simulink model "Battery_module"  (R2021a)
settings: Solver=VariableStepAuto  StartTime=0.0  StopTime=1.5  RelTol=1e-3
undefined symbols (not defined in the file or in its folder): Ion, Lithium
libraries: spsOnDelayLib x2, spsBatteryLib x2, spsDCVoltageSourceLib x1, spsSeriesRLCBranchLib x1, pid_lib x1, eePwmGenerator x1, spsMeanLib x1, spsUniversalBridgeLib x1, spsVoltageMeasurementLib x1, spspowerguiLib x1, SignalEditorBlockLib x1
settings Model: Creator=XieWHirlwind_TB  LastModifiedBy=XieWHirlwind_TB

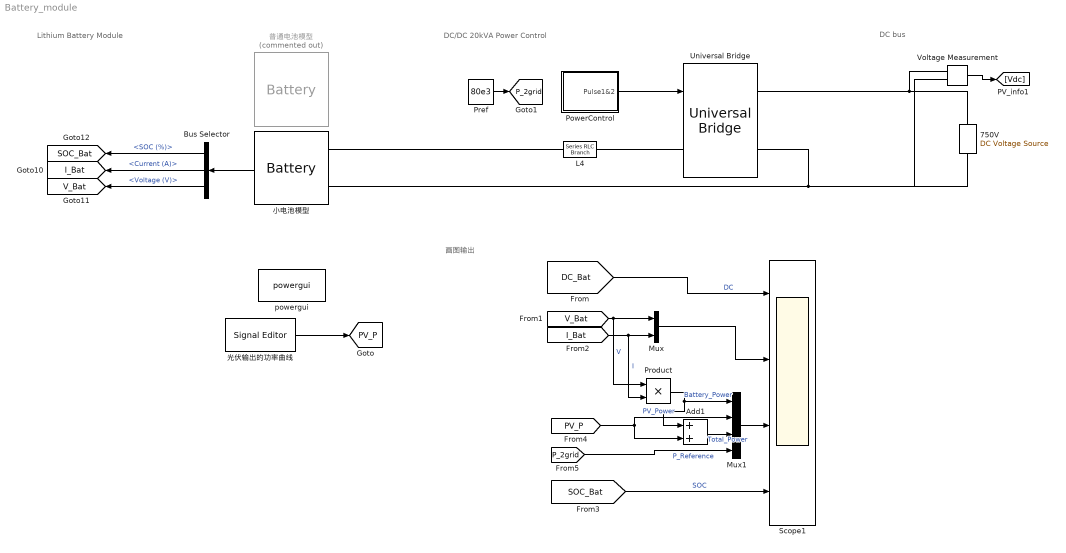
== system Battery_module ==
  note: 画图输出
  note: DC/DC 20kVA Power Control
  note: Lithium Battery Module
  note: DC bus
  750V : spsDCVoltageSourceLib/DC Voltage Source  Amplitude=750  Measurements=None
  Add1 : Sum
  Bus Selector : BusSelector  OutputSignals=SOC (%),Current (A),Voltage (V)
  L4 : spsSeriesRLCBranchLib/Series RLC Branch  LConnTagsString=__new0  RConnTagsString=__new0  BranchType=RL  Resistance=0.001  Inductance=1e-3  SetiL0=off  InitialCurrent=0  Capacitance=1e-6  Setx0=off  InitialVoltage=0  Measurements=None
  Mux : Mux  Inputs=2
  Mux1 : Mux
  PowerControl : Subsystem
  Pref : Constant  Value=80e3
  Product : Product
  Scope1 : Scope  NumInputPorts=4
  Universal Bridge : spsUniversalBridgeLib/Universal Bridge  Arms=1  SnubberResistance=1e5  SnubberCapacitance=inf  Device=IGBT / Diodes  Ron=1e-3  Lon=0  ForwardVoltages="[0.7  0.7]"  ForwardVoltage=0  GTOparameters=[ 10e-6 , 20e-6 ]  IGBTparameters=[ 1e-6 , 2e-6 ]  Measurements=None  Measurements_2=None  converterType=Rectifier
  Voltage Measurement : spsVoltageMeasurementLib/Voltage Measurement  PhasorSimulation=off  OutputType=Complex  PSBequivalent=0
  powergui : spspowerguiLib/powergui  Priority=1  SimulationMode=Discrete  SampleTime=2e-6  frequency=60  Iterations=50  frequencyindice=0  Pbase=100e6  ErrMax=1e-4  UnitsV=kV  UnitsW=MW  buscounter=0  FunctionMessages=off  echomessages=off  EnableUseOfTLC=off  CurrentSourceSwitches=off  DisableSnubberDevices=off  DisableRonSwitches=off  DisableVfSwitches=off  DisplayEquations=off  AutomaticDiscreteSolvers=off  SolverType=Tustin/Backward Euler (TBE)  Interpol=off  ExternalGateDelay=off  methode=off  Ts=100  x0status=blocks  SPID=on  SwTol=0  HookPort=off  NonlinearTolerance=1e-4  nMaxIteration=100  ContinueOnMaxIteration=off  RestoreLinks=warning  ResistiveCurrentMeasurement=off  Frange=[0:2:500]  Ylog=off  Xlog=on  ShowGrid=off  save=off  variable=ZData  structure=0  ZoomFFT=off  StartTime=0.0  cycles=1  DisplayStyle=1  fundamental=60  FreqAxis=off  MaxFrequency=1000  frequencyindicesteady=1  RmsSteady=1  display=off
  光伏输出的功率曲线 : SignalEditorBlockLib/Signal Editor  FileName=PV_Power_1.mat  ActiveScenario=InRatedPower  ActiveSignal=PV_Power  IsBus=off  OutputBusObjectStr=Bus: BusObject  SampleTime=0  ZeroCross=off  OutputAfterFinalValue=Setting to zero  Unit=inherit  PreserveSignalName=on
  小电池模型 : spsBatteryLib/Battery  BatType=Lithium-Ion  ShowTempParam=off  ThermalPreset=no  ShowAgeParam=off  NomV=640  NomQ=62.5/1000  SOC=50  Batt_Tr=30  PresetModel=off  MaxQ=62.5/100000  MinV=480  FullV=744.9518  Dis_rate=27.1739  R=0.1024  Normal_OP=56.5217/100000  expZone="[691.4469      3.070652/100000]"  current=[6.5 13 32.5]  Units=Time  Tci=20  NomT=20  T2=-30  MaxQ2=4.8  FullV2=7.1  Normal_OP2=5.655  expZone2="[6.58           1]"  Rca=0.6  ti=2000  Dp=0  Neq0=0  Tsim=1e6  Ta1=25  Qeol=5.4*0.9  Reol=0.013333*1.2  Char_age=[2.3478, 3]  Dis_age=[2.3478, 10]  N1=1500  N2=10500  N3=1000  N4=1400  Ta2=45  N5=950
  普通电池模型 : spsBatteryLib/Battery  Commented=on  BatType=Lithium-Ion  ShowTempParam=off  ThermalPreset=no  ShowAgeParam=off  NomV=640  NomQ=62.5  SOC=50  Batt_Tr=30  PresetModel=on  MaxQ=62.5  MinV=480  FullV=744.9518  Dis_rate=27.1739  R=0.1024  Normal_OP=56.5217  expZone="[691.4469      3.070652]"  current=[6.5 13 32.5]  Units=Time  Tci=20  NomT=20  T2=-30  MaxQ2=4.8  FullV2=7.1  Normal_OP2=5.655  expZone2="[6.58           1]"  Rca=0.6  ti=2000  Dp=0  Neq0=0  Tsim=1e6  Ta1=25  Qeol=5.4*0.9  Reol=0.013333*1.2  Char_age=[2.3478, 3]  Dis_age=[2.3478, 10]  N1=1500  N2=10500  N3=1000  N4=1400  Ta2=45  N5=950
  tag scope: I_Bat=global, PV_P=global, P_2grid=global, SOC_Bat=global, V_Bat=global
  wires:
  Bus Selector/3 -> [V_Bat]  "<Voltage (V)>"
  小电池模型/1 -> Bus Selector/1
  Bus Selector/1 -> [SOC_Bat]  "<SOC (%)>"
  Bus Selector/2 -> [I_Bat]  "<Current (A)>"
  Voltage Measurement/1 -> [Vdc]
  光伏输出的功率曲线/1 -> [PV_P]
  [DC_Bat] -> Scope1/1  "DC"
  [V_Bat] -> Mux/1, Product/1  "V"
  [I_Bat] -> Product/2, Mux/2  "I"
  [SOC_Bat] -> Scope1/4  "SOC"
  Mux/1 -> Scope1/2
  [PV_P] -> Add1/2, Mux1/2  "PV_Power"
  Mux1/1 -> Scope1/3
  Product/1 -> Add1/1, Mux1/1  "Battery_Power"
  Add1/1 -> Mux1/3  "Total_Power"
  PowerControl/1(Pulse1&2) -> Universal Bridge/1
  Pref/1 -> [P_2grid]
  [P_2grid] -> Mux1/4  "P_Reference"
  connections:
  750V/LConn1 -- Voltage Measurement/LConn2 -- 小电池模型/LConn2 -- Universal Bridge/RConn2
  Universal Bridge/LConn1 -- L4/RConn1
  小电池模型/LConn1 -- L4/LConn1
  Universal Bridge/RConn1 -- 750V/RConn1 -- Voltage Measurement/LConn1

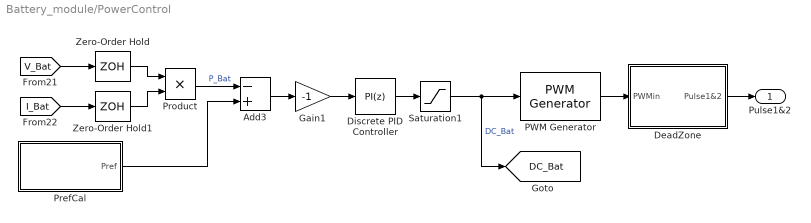
== system Battery_module/PowerControl ==
  Add3 : Sum  Inputs=-+
  DeadZone : Subsystem
  Discrete PID Controller : pid_lib/PID Controller  Controller=PI  Form=Parallel  TimeDomain=Discrete-time  UseExternalTs=off  SampleTime=1e-4  IntegratorMethod=Forward Euler  FilterMethod=Forward Euler  ControllerParametersSource=internal  P=2e-6  I=2e-3  D=0  UseFilter=on  N=100  TunerSelectOption=Transfer Function Based (PID Tuner App)  InitialConditionSource=internal  InitialConditionForIntegrator=0.8  InitialConditionForFilter=0  DifferentiatorICPrevScaledInput=0  ExternalReset=none  TrackingMode=off  Kt=1  LimitOutput=off  SatLimitsSource=internal  UpperSaturationLimit=1  LowerSaturationLimit=0  LinearizeAsGain=off  AntiWindupMode=none  Kb=1  POutMin=[]  POutMax=[]  IOutMin=[]  IOutMax=[]  DOutMin=[]  DOutMax=[]  NOutMin=[]  NOutMax=[]  SumOutMin=[]  SumOutMax=[]  SaturationOutMin=[]  SaturationOutMax=[]  PParamMin=[]  PParamMax=[]  IParamMin=[]  IParamMax=[]  DParamMin=[]  DParamMax=[]  NParamMin=[]  NParamMax=[]  KbParamMin=[]  KbParamMax=[]  KtParamMin=[]  KtParamMax=[]  KbOutMin=[]  KbOutMax=[]  KtOutMin=[]  KtOutMax=[]  IntegratorOutMin=[]  IntegratorOutMax=[]  FilterOutMin=[]  FilterOutMax=[]  SumI1OutMin=[]  SumI1OutMax=[]  SumI2OutMin=[]  SumI2OutMax=[]  SumI3OutMin=[]  SumI3OutMax=[]  SumI4OutMin=[]  SumI4OutMax=[]  SumDOutMin=[]  SumDOutMax=[]  DifferentiatorOutMin=[]  DifferentiatorOutMax=[]  FilterDiffOutCoefMin=[]  FilterDiffOutCoefMax=[]  ReciprocalOutMin=[]  ReciprocalOutMax=[]  SumDenOutMin=[]  SumDenOutMax=[]  SumNumOutMin=[]  SumNumOutMax=[]  DivideOutMin=[]  DivideOutMax=[]  UdiffTsProdOutMin=[]  UdiffTsProdOutMax=[]  NTsProdOutMin=[]  NTsProdOutMax=[]  UintegralTsProdOutMin=[]  UintegralTsProdOutMax=[]  UngainTsProdOutMin=[]  UngainTsProdOutMax=[]  IntegratorContinuousStateAttributes=''  IntegratorStateMustResolveToSignalObject=off  IntegratorRTWStateStorageClass=Auto  FilterContinuousStateAttributes=''  FilterStateMustResolveToSignalObject=off  FilterRTWStateStorageClass=Auto  ParallelPVariant=InternalParameters  IdealPVariant=Disabled  IVariant=InternalParameters  DVariant=Disabled  IntegratorVariant=Discrete  SatVariant=Disabled  AWVariant=Passthrough  PCopyVariant=Disabled  TRVariant=Disabled  FdbkBlocksVariant=Forward  IdealPFdbkVariant=Disabled  SatFdbkVariant=Disabled  DerivativeFilterVariant=Disabled  NVariant=Disabled  NCopyVariant=Disabled_SignalSpec  FilterICVariant=Disabled  IntegratorICVariant=InternalICs  ExternalResetVariant=Disabled  TRSumVariant=Passthrough  SumFdbkVariant=Disabled  SumVariant=Sum_PI  TsampFilterVariant=InternalTs  TsampNgainVariant=Passthrough  TsampIntegralVariant=Passthrough  ExternalSaturationOutDataTypeStr=Inherit: Same as second input
  Gain1 : Gain  Gain=-1
  PWM Generator : eePwmGenerator/PWM Generator  CarrCount=Up  Tper=1e-4  Ts=2e-6
  PrefCal : Subsystem
  Product : Product
  Saturation1 : Saturate  UpperLimit=0.98  LowerLimit=0
  Zero-Order Hold : ZeroOrderHold  SampleTime=1e-4
  Zero-Order Hold1 : ZeroOrderHold  SampleTime=1e-4
  Pulse1&2 : Outport
  tag scope: DC_Bat=global
  wires:
  Zero-Order Hold1/1 -> Product/2
  Zero-Order Hold/1 -> Product/1
  Gain1/1 -> Discrete PID Controller/1
  Add3/1 -> Gain1/1
  Saturation1/1 -> PWM Generator/1, [DC_Bat]  "DC_Bat"
  Discrete PID Controller/1 -> Saturation1/1
  Product/1 -> Add3/1  "P_Bat"
  [I_Bat] -> Zero-Order Hold1/1
  [V_Bat] -> Zero-Order Hold/1
  PWM Generator/1 -> DeadZone/1(PWMin)
  DeadZone/1(Pulse1&2) -> Pulse1&2/1
  PrefCal/1(Pref) -> Add3/2

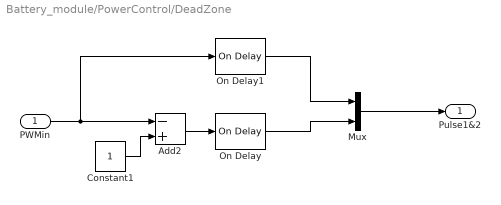
== system Battery_module/PowerControl/DeadZone ==
  PWMin : Inport
  Add2 : Sum  Inputs=-+
  Constant1 : Constant
  Mux : Mux  Inputs=2
  On Delay : spsOnDelayLib/On Delay  DelayType=On delay  delay=2e-6  ic=0  Ts=0
      settings: SourceProductBaseCode=PS
  On Delay1 : spsOnDelayLib/On Delay  DelayType=On delay  delay=2e-6  ic=0  Ts=0
      settings: SourceProductBaseCode=PS
  Pulse1&2 : Outport
  wires:
  Constant1/1 -> Add2/2
  PWMin/1 -> Add2/1, On Delay1/1
  Add2/1 -> On Delay/1
  Mux/1 -> Pulse1&2/1
  On Delay1/1 -> Mux/1
  On Delay/1 -> Mux/2

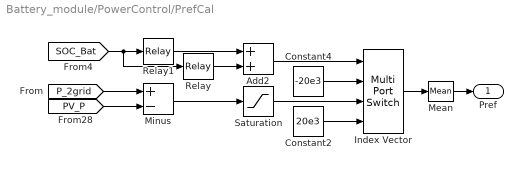
== system Battery_module/PowerControl/PrefCal ==
  Add2 : Sum
  Constant2 : Constant  Value=20e3
  Constant4 : Constant  Value=-20e3
  Index Vector : MultiPortSwitch  DataPortOrder=Zero-based contiguous  zeroidx=on
  Mean : spsMeanLib/Mean  Freq=1e4  Vinit=0  Ts=2e-6
  Minus : Sum  Inputs=+-
  Relay : Relay  OnSwitchValue=30  OffSwitchValue=10
  Relay1 : Relay  OnSwitchValue=90  OffSwitchValue=70
  Saturation : Saturate  UpperLimit=20e3  LowerLimit=-20e3
  Pref : Outport
  wires:
  Add2/1 -> Index Vector/1
  Saturation/1 -> Index Vector/3
  Minus/1 -> Saturation/1
  Index Vector/1 -> Mean/1
  [SOC_Bat] -> Relay/1, Relay1/1
  Relay/1 -> Add2/2
  Relay1/1 -> Add2/1
  Constant2/1 -> Index Vector/4
  Constant4/1 -> Index Vector/2
  [P_2grid] -> Minus/1
  [PV_P] -> Minus/2
  Mean/1 -> Pref/1
